simulink model "pc_375"  (R2014a)
settings: Solver=FixedStepDiscrete  StartTime=0.0  StopTime=inf  RelTol=1e-3
libraries: amg_usbconverter_n_connect_lib x5
settings Model: Creator=lenovo  LastModifiedBy=lenovo

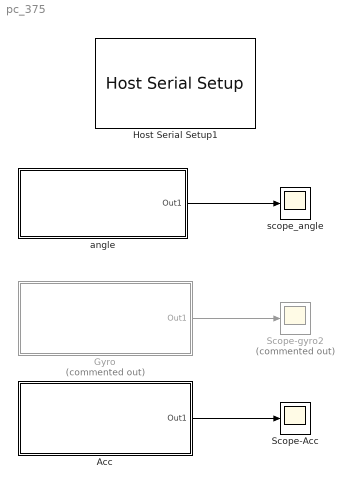
== system pc_375 ==
  Acc : Subsystem
  Gyro : Subsystem  Commented=on
  Host Serial Setup1 : amg_usbconverter_n_connect_lib/Host Serial Setup  conf=setup  port=<auto>  baudrate=115200  databits=8  parity=None  stopbit=1  flowcontrol=None  transfer=Blocking  timeout=2  packetmode=Binary  initialvalues=[]  binheader='7E 7E'  binterminator='03 03'  porttype_double=0  porttype_single=1  porttype_int8=0  porttype_uint8=0  porttype_int16=0  porttype_uint16=0  porttype_int32=0  porttype_uint32=2  asciiformat='%d %u %x'  rx_asciiterminator="CRLF (0x0D 0x0A - \"\\r\\n\")"  tx_asciiterminator="CRLF (0x0D 0x0A - \"\\r\\n\")"  sampletime=1/204  enablecustomportlabel=off  cinputportlabel=0  coutputportlabel=A  portpinstr=0  blockid=HostSerialSetup1  inputporttype=[]  inputportwidth=[]  inputportlabel={}  outputporttype=[]  outputportwidth=[]  outputportlabel={}  compat=0  optionstring=[]  autoport='COM4'
  Scope-Acc : Scope
      settings: TimeRange=10  YMin=-1.05  YMax=0.05
  Scope-gyro2 : Scope  Commented=on
      settings: TimeRange=10  YMin=-27.5  YMax=2.5  SaveName=ScopeData3
  angle : Subsystem
  scope_angle : Scope
      settings: TimeRange=10  YMin=0  YMax=15
  wires:
  Gyro/1(Out1) -> Scope-gyro2/1
  angle/1(Out1) -> scope_angle/1
  Acc/1(Out1) -> Scope-Acc/1

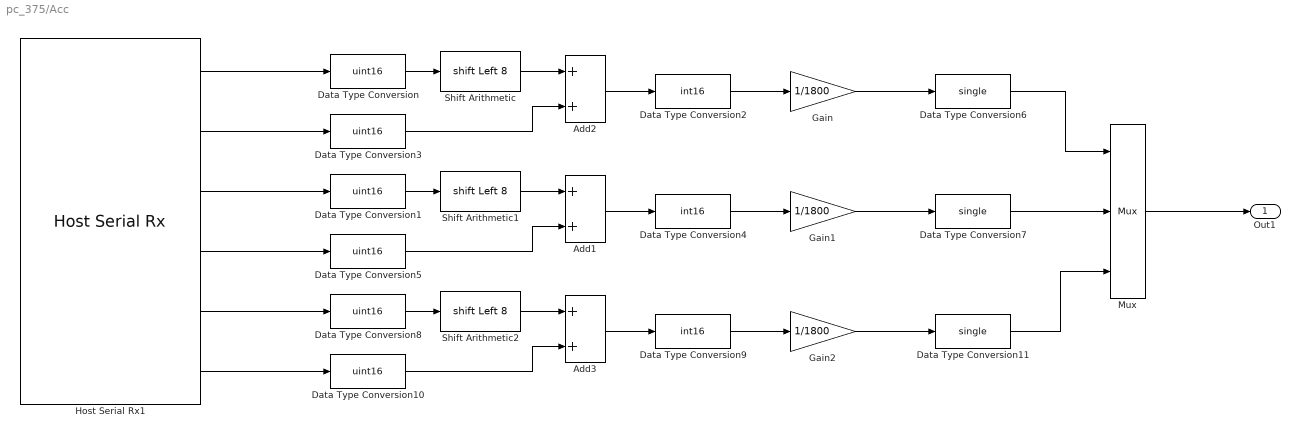
== system pc_375/Acc ==
  Add1 : Sum
  Add2 : Sum
  Add3 : Sum
  Data Type Conversion{,1,3,5,8,10} (6 alike) : DataTypeConversion  OutDataTypeStr=uint16
  Data Type Conversion11 : DataTypeConversion  OutDataTypeStr=single
  Data Type Conversion2 : DataTypeConversion  OutDataTypeStr=int16
  Data Type Conversion4 : DataTypeConversion  OutDataTypeStr=int16
  Data Type Conversion6 : DataTypeConversion  OutDataTypeStr=single
  Data Type Conversion7 : DataTypeConversion  OutDataTypeStr=single
  Data Type Conversion9 : DataTypeConversion  OutDataTypeStr=int16
  Gain : Gain  Gain=1/1800
  Gain1 : Gain  Gain=1/1800
  Gain2 : Gain  Gain=1/1800
  Host Serial Rx1 : amg_usbconverter_n_connect_lib/Host Serial Rx  conf=rx  port=<auto>  baudrate=115200  databits=8  parity=None  stopbit=1  flowcontrol=None  transfer=Blocking  timeout=5  packetmode=Binary  enableinitialvalues=off  initialvalues=[]  binheader='ff fa'  binterminator='0d 0a'  porttype_double=0  porttype_single=0  porttype_int8=0  porttype_uint8=6  porttype_int16=0  porttype_uint16=0  porttype_int32=0  porttype_uint32=0  asciiformat='%d,%f'  rx_asciiterminator="CRLF (0x0D 0x0A - \"\\r\\n\")"  tx_asciiterminator="CRLF (0x0D 0x0A - \"\\r\\n\")"  sampletime=-1  enablecustomportlabel=off  cinputportlabel=0  coutputportlabel=A  portpinstr=0  blockid=AccHostSerialRx1  inputporttype=[]  inputportwidth=[]  inputportlabel={}  outputporttype=[3 3 3 3 3 3]  outputportwidth=[1 1 1 1 1 1]  outputportlabel={'uint8','uint8','uint8','uint8','uint8','uint8'}  compat=0  optionstring=[]  autoport='COM4'
  Mux : Mux  Inputs=3
  Shift Arithmetic : ArithShift  BitShiftNumber=8  BitShiftDirection=Left
  Shift Arithmetic1 : ArithShift  BitShiftNumber=8  BitShiftDirection=Left
  Shift Arithmetic2 : ArithShift  BitShiftNumber=8  BitShiftDirection=Left
  Out1 : Outport
  wires:
  Host Serial Rx1/5 -> Data Type Conversion8/1
  Host Serial Rx1/3 -> Data Type Conversion1/1
  Host Serial Rx1/6 -> Data Type Conversion10/1
  Host Serial Rx1/4 -> Data Type Conversion5/1
  Host Serial Rx1/2 -> Data Type Conversion3/1
  Host Serial Rx1/1 -> Data Type Conversion/1
  Data Type Conversion2/1 -> Gain/1
  Data Type Conversion10/1 -> Add3/2
  Data Type Conversion7/1 -> Mux/2
  Shift Arithmetic1/1 -> Add1/1
  Gain2/1 -> Data Type Conversion11/1
  Gain1/1 -> Data Type Conversion7/1
  Data Type Conversion1/1 -> Shift Arithmetic1/1
  Add1/1 -> Data Type Conversion4/1
  Shift Arithmetic2/1 -> Add3/1
  Data Type Conversion9/1 -> Gain2/1
  Gain/1 -> Data Type Conversion6/1
  Data Type Conversion3/1 -> Add2/2
  Add3/1 -> Data Type Conversion9/1
  Add2/1 -> Data Type Conversion2/1
  Data Type Conversion6/1 -> Mux/1
  Data Type Conversion11/1 -> Mux/3
  Shift Arithmetic/1 -> Add2/1
  Data Type Conversion/1 -> Shift Arithmetic/1
  Mux/1 -> Out1/1
  Data Type Conversion4/1 -> Gain1/1
  Data Type Conversion5/1 -> Add1/2
  Data Type Conversion8/1 -> Shift Arithmetic2/1

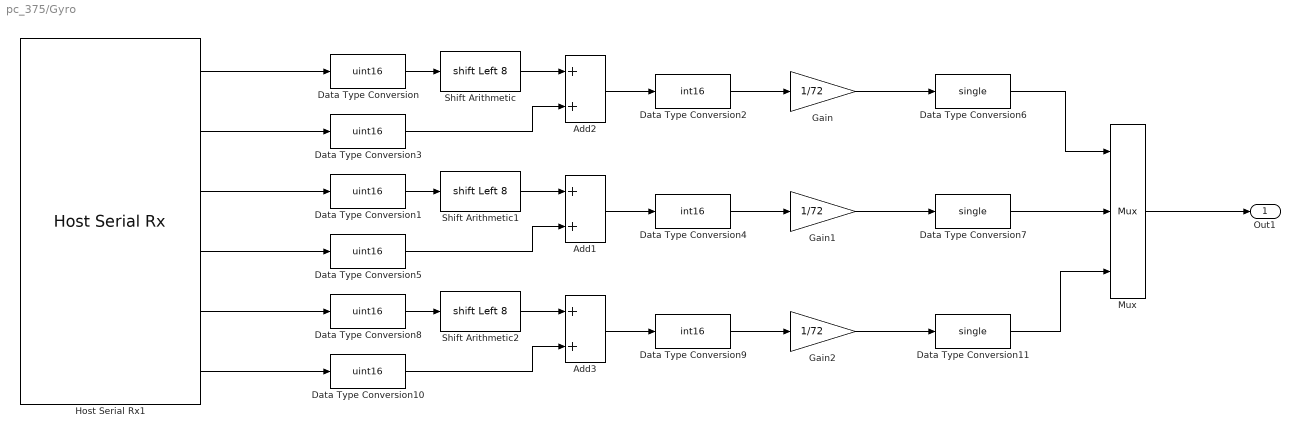
== system pc_375/Gyro ==
  Add1 : Sum
  Add2 : Sum
  Add3 : Sum
  Data Type Conversion{,1,3,5,8,10} (6 alike) : DataTypeConversion  OutDataTypeStr=uint16
  Data Type Conversion11 : DataTypeConversion  OutDataTypeStr=single
  Data Type Conversion2 : DataTypeConversion  OutDataTypeStr=int16
  Data Type Conversion4 : DataTypeConversion  OutDataTypeStr=int16
  Data Type Conversion6 : DataTypeConversion  OutDataTypeStr=single
  Data Type Conversion7 : DataTypeConversion  OutDataTypeStr=single
  Data Type Conversion9 : DataTypeConversion  OutDataTypeStr=int16
  Gain : Gain  Gain=1/72
  Gain1 : Gain  Gain=1/72
  Gain2 : Gain  Gain=1/72
  Host Serial Rx1 : amg_usbconverter_n_connect_lib/Host Serial Rx  conf=rx  port=COM4  baudrate=115200  databits=8  parity=None  stopbit=1  flowcontrol=None  transfer=Blocking  timeout=5  packetmode=Binary  enableinitialvalues=off  initialvalues=[]  binheader='ff fb'  binterminator='fb ff'  porttype_double=0  porttype_single=0  porttype_int8=0  porttype_uint8=6  porttype_int16=0  porttype_uint16=0  porttype_int32=0  porttype_uint32=0  asciiformat='%d,%f'  rx_asciiterminator="CRLF (0x0D 0x0A - \"\\r\\n\")"  tx_asciiterminator="CRLF (0x0D 0x0A - \"\\r\\n\")"  sampletime=-1  enablecustomportlabel=off  cinputportlabel=0  coutputportlabel=A  portpinstr=0  blockid=GyroHostSerialRx1  inputporttype=[]  inputportwidth=[]  inputportlabel={}  outputporttype=[3 3 3 3 3 3]  outputportwidth=[1 1 1 1 1 1]  outputportlabel={'uint8','uint8','uint8','uint8','uint8','uint8'}  compat=0  optionstring=[]  autoport='COM4'
  Mux : Mux  Inputs=3
  Shift Arithmetic : ArithShift  BitShiftNumber=8  BitShiftDirection=Left
  Shift Arithmetic1 : ArithShift  BitShiftNumber=8  BitShiftDirection=Left
  Shift Arithmetic2 : ArithShift  BitShiftNumber=8  BitShiftDirection=Left
  Out1 : Outport
  wires:
  Host Serial Rx1/5 -> Data Type Conversion8/1
  Host Serial Rx1/3 -> Data Type Conversion1/1
  Host Serial Rx1/6 -> Data Type Conversion10/1
  Host Serial Rx1/4 -> Data Type Conversion5/1
  Host Serial Rx1/2 -> Data Type Conversion3/1
  Host Serial Rx1/1 -> Data Type Conversion/1
  Data Type Conversion2/1 -> Gain/1
  Data Type Conversion10/1 -> Add3/2
  Data Type Conversion7/1 -> Mux/2
  Shift Arithmetic1/1 -> Add1/1
  Gain2/1 -> Data Type Conversion11/1
  Gain1/1 -> Data Type Conversion7/1
  Data Type Conversion1/1 -> Shift Arithmetic1/1
  Add1/1 -> Data Type Conversion4/1
  Shift Arithmetic2/1 -> Add3/1
  Data Type Conversion9/1 -> Gain2/1
  Gain/1 -> Data Type Conversion6/1
  Data Type Conversion3/1 -> Add2/2
  Add3/1 -> Data Type Conversion9/1
  Add2/1 -> Data Type Conversion2/1
  Data Type Conversion6/1 -> Mux/1
  Data Type Conversion11/1 -> Mux/3
  Shift Arithmetic/1 -> Add2/1
  Data Type Conversion/1 -> Shift Arithmetic/1
  Mux/1 -> Out1/1
  Data Type Conversion4/1 -> Gain1/1
  Data Type Conversion5/1 -> Add1/2
  Data Type Conversion8/1 -> Shift Arithmetic2/1

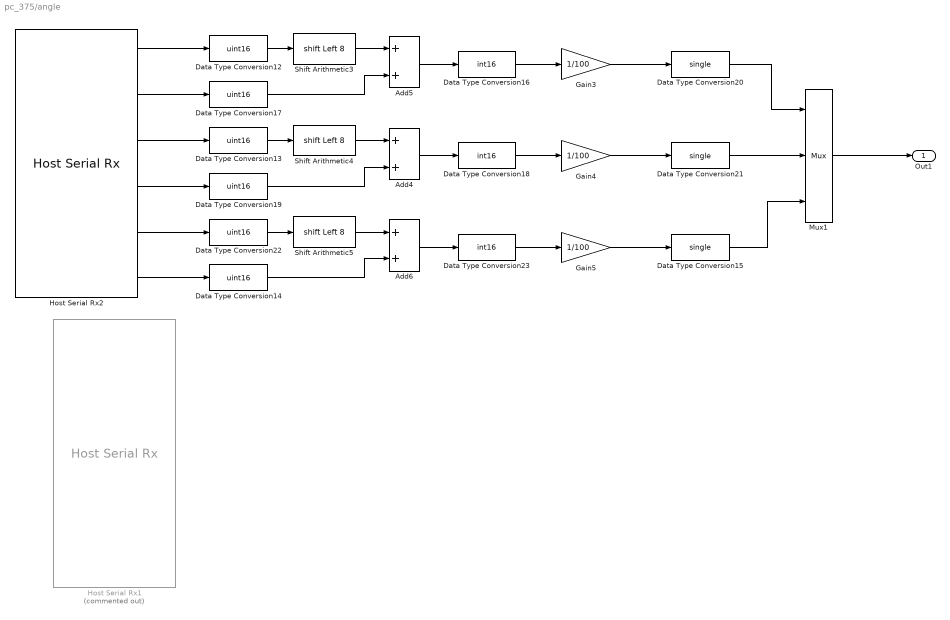
== system pc_375/angle ==
  Add4 : Sum
  Add5 : Sum
  Add6 : Sum
  Data Type Conversion{12..14,17,19,22} (6 alike) : DataTypeConversion  OutDataTypeStr=uint16
  Data Type Conversion15 : DataTypeConversion  OutDataTypeStr=single
  Data Type Conversion16 : DataTypeConversion  OutDataTypeStr=int16
  Data Type Conversion18 : DataTypeConversion  OutDataTypeStr=int16
  Data Type Conversion20 : DataTypeConversion  OutDataTypeStr=single
  Data Type Conversion21 : DataTypeConversion  OutDataTypeStr=single
  Data Type Conversion23 : DataTypeConversion  OutDataTypeStr=int16
  Gain3 : Gain  Gain=1/100
  Gain4 : Gain  Gain=1/100
  Gain5 : Gain  Gain=1/100
  Host Serial Rx1 : amg_usbconverter_n_connect_lib/Host Serial Rx  Commented=on  conf=rx  port=<auto>  baudrate=115200  databits=8  parity=None  stopbit=1  flowcontrol=None  transfer=Blocking  timeout=5  packetmode=Binary  enableinitialvalues=off  initialvalues=[]  binheader='ff fb'  binterminator=''  porttype_double=0  porttype_single=0  porttype_int8=0  porttype_uint8=6  porttype_int16=0  porttype_uint16=0  porttype_int32=0  porttype_uint32=0  asciiformat='%d,%f'  rx_asciiterminator="CRLF (0x0D 0x0A - \"\\r\\n\")"  tx_asciiterminator="CRLF (0x0D 0x0A - \"\\r\\n\")"  sampletime=-1  enablecustomportlabel=off  cinputportlabel=0  coutputportlabel=A  portpinstr=0  blockid=angleHostSerialRx1  inputporttype=[]  inputportwidth=[]  inputportlabel={}  outputporttype=[3 3 3 3 3 3]  outputportwidth=[1 1 1 1 1 1]  outputportlabel={'uint8','uint8','uint8','uint8','uint8','uint8'}  compat=0  optionstring=[]  autoport='COM4'
  Host Serial Rx2 : amg_usbconverter_n_connect_lib/Host Serial Rx  conf=rx  port=<auto>  baudrate=115200  databits=8  parity=None  stopbit=1  flowcontrol=None  transfer=Blocking  timeout=5  packetmode=Binary  enableinitialvalues=off  initialvalues=[]  binheader='ff fc'  binterminator='0d 0a'  porttype_double=0  porttype_single=0  porttype_int8=0  porttype_uint8=6  porttype_int16=0  porttype_uint16=0  porttype_int32=0  porttype_uint32=0  asciiformat='%d,%f'  rx_asciiterminator="CRLF (0x0D 0x0A - \"\\r\\n\")"  tx_asciiterminator="CRLF (0x0D 0x0A - \"\\r\\n\")"  sampletime=-1  enablecustomportlabel=off  cinputportlabel=0  coutputportlabel=A  portpinstr=0  blockid=angleHostSerialRx2  inputporttype=[]  inputportwidth=[]  inputportlabel={}  outputporttype=[3 3 3 3 3 3]  outputportwidth=[1 1 1 1 1 1]  outputportlabel={'uint8','uint8','uint8','uint8','uint8','uint8'}  compat=0  optionstring=[]  autoport='COM4'
  Mux1 : Mux  Inputs=3
  Shift Arithmetic3 : ArithShift  BitShiftNumber=8  BitShiftDirection=Left
  Shift Arithmetic4 : ArithShift  BitShiftNumber=8  BitShiftDirection=Left
  Shift Arithmetic5 : ArithShift  BitShiftNumber=8  BitShiftDirection=Left
  Out1 : Outport
  wires:
  Host Serial Rx2/6 -> Data Type Conversion14/1
  Host Serial Rx2/1 -> Data Type Conversion12/1
  Host Serial Rx2/5 -> Data Type Conversion22/1
  Host Serial Rx2/2 -> Data Type Conversion17/1
  Host Serial Rx2/3 -> Data Type Conversion13/1
  Host Serial Rx2/4 -> Data Type Conversion19/1
  Data Type Conversion16/1 -> Gain3/1
  Shift Arithmetic4/1 -> Add4/1
  Data Type Conversion23/1 -> Gain5/1
  Data Type Conversion12/1 -> Shift Arithmetic3/1
  Shift Arithmetic5/1 -> Add6/1
  Shift Arithmetic3/1 -> Add5/1
  Data Type Conversion15/1 -> Mux1/3
  Data Type Conversion18/1 -> Gain4/1
  Mux1/1 -> Out1/1
  Gain5/1 -> Data Type Conversion15/1
  Gain3/1 -> Data Type Conversion20/1
  Data Type Conversion19/1 -> Add4/2
  Data Type Conversion14/1 -> Add6/2
  Data Type Conversion22/1 -> Shift Arithmetic5/1
  Add4/1 -> Data Type Conversion18/1
  Gain4/1 -> Data Type Conversion21/1
  Data Type Conversion17/1 -> Add5/2
  Add5/1 -> Data Type Conversion16/1
  Add6/1 -> Data Type Conversion23/1
  Data Type Conversion21/1 -> Mux1/2
  Data Type Conversion20/1 -> Mux1/1
  Data Type Conversion13/1 -> Shift Arithmetic4/1
